simulink model "c_sim"  (R2026a)
settings: Solver=ode4  StopTime=600  FixedStep=1.0
libraries: simulink x2
settings Model: Creator=honda  LastModifiedBy=honda

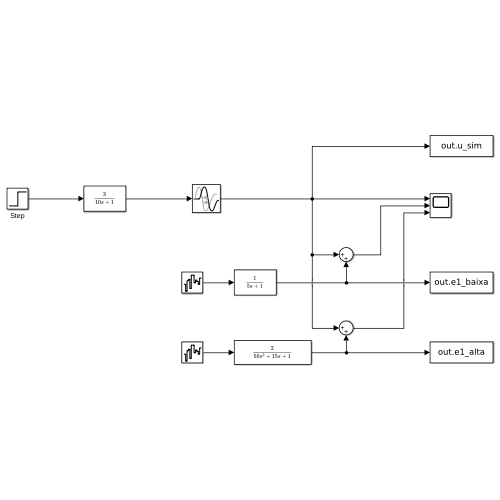
[thumbnail: Simulink's stored preview of the top-level diagram]
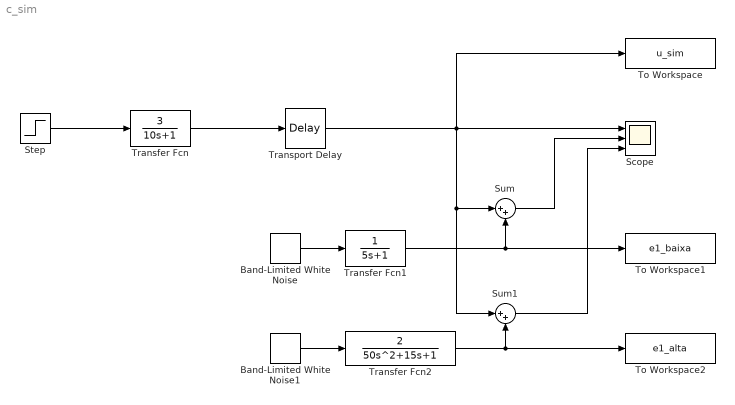
== system c_sim ==
  Band-Limited White Noise : simulink/Sources/Band-Limited White Noise  Cov=[0.0001]  Ts=1  seed=[12345]
  Band-Limited White Noise1 : simulink/Sources/Band-Limited White Noise  Cov=[0.01]  Ts=1  seed=[23341]
  Scope : Scope  NumInputPorts=3
      settings: ActiveDisplayYMinimum=-0.19469103451799066  ActiveDisplayYMaximum=0.53048690385299657  DataLoggingVariableName=y
  Step : Step  Time=275  FinalValue=0.1  SampleTime=0
  Sum : Sum  Inputs=|++
  Sum1 : Sum  Inputs=|++
  To Workspace : ToWorkspace  VariableName=u_sim  SampleTime=1
  To Workspace1 : ToWorkspace  VariableName=e1_baixa  SampleTime=1
  To Workspace2 : ToWorkspace  VariableName=e1_alta  SampleTime=1
  Transfer Fcn : TransferFcn  Numerator=[3]  Denominator=[10 1]
  Transfer Fcn1 : TransferFcn  Denominator=[5 1]
  Transfer Fcn2 : TransferFcn  Numerator=[2]  Denominator=[50 15 1]
  Transport Delay : TransportDelay  DelayTime=5
  wires:
  Step/1 -> Transfer Fcn/1
  Transfer Fcn/1 -> Transport Delay/1
  Transport Delay/1 -> Scope/1, Sum1/1, Sum/1, To Workspace/1
  Band-Limited White Noise/1 -> Transfer Fcn1/1
  Transfer Fcn1/1 -> To Workspace1/1, Sum/2
  Sum/1 -> Scope/2
  Band-Limited White Noise1/1 -> Transfer Fcn2/1
  Transfer Fcn2/1 -> To Workspace2/1, Sum1/2
  Sum1/1 -> Scope/3
